simulink model "gyroYawLoop"  (R2015a)
settings: Solver=ode45  StartTime=0.0  StopTime=10  RelTol=1e-3
undefined symbols (not defined in the file or in its folder): dt, plantTorqueOffset, torqueOffset
libraries: simulink x1, vrlib x1
settings Model: Creator=johnz  LastModifiedBy=johnz

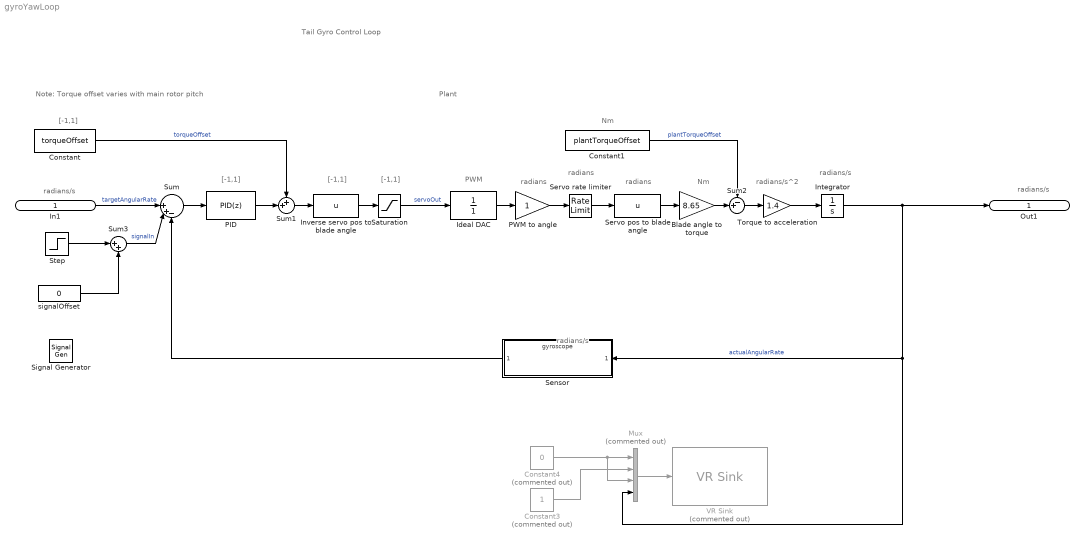
== system gyroYawLoop ==
  note: Tail Gyro Control Loop
  note: Note: Torque offset varies with main rotor pitch
  note: Plant
  note: [-1,1]
  note: radians/s
  note: radians
  note: radians/s^2
  note: radians/s
  note: [-1,1]
  note: [-1,1]
  note: [-1,1]
  note: Nm
  note: radians/s
  note: Nm
  note: radians
  note: radians
  note: radians/s
  note: PWM
  In1 : Inport  SampleTime=dt
  Blade angle to torque : Gain  Gain=8.65
  Constant : Constant  Value=torqueOffset  SampleTime=dt
  Constant1 : Constant  Value=plantTorqueOffset
  Constant3 : Constant  Commented=on
  Constant4 : Constant  Commented=on  Value=0
  Ideal DAC : TransferFcn  Denominator=[1]
  Integrator : Integrator
  "Inverse servo pos to blade angle " : Fcn  Expr=u
  Mux : Mux  Commented=on
  PID : simulink/Continuous/PID Controller  Controller=PID  TimeDomain=Discrete-time  SampleTime=dt  IntegratorMethod=Forward Euler  FilterMethod=Forward Euler  Form=Parallel  UseFilter=off  ControllerParametersSource=internal  P=1.08315527025018  I=2.38693404249782  D=.035  N=100  InitialConditionSource=internal  InitialConditionForIntegrator=0  InitialConditionForFilter=0  ExternalReset=none  ZeroCross=off  LimitOutput=on  UpperSaturationLimit=1 - torqueOffset  LowerSaturationLimit=-1 - torqueOffset  LinearizeAsGain=on  AntiWindupMode=clamping  Kb=0.5  TrackingMode=off  Kt=1  PParamMin=[]  PParamMax=[]  IParamMin=[]  IParamMax=[]  DParamMin=[]  DParamMax=[]  NParamMin=[]  NParamMax=[]  KbParamMin=[]  KbParamMax=[]  KtParamMin=[]  KtParamMax=[]  POutMin=[]  POutMax=[]  IOutMin=[]  IOutMax=[]  DOutMin=[]  DOutMax=[]  NOutMin=[]  NOutMax=[]  KbOutMin=[]  KbOutMax=[]  KtOutMin=[]  KtOutMax=[]  IntegratorOutMin=[]  IntegratorOutMax=[]  FilterOutMin=[]  FilterOutMax=[]  SumOutMin=[]  SumOutMax=[]  SumI1OutMin=[]  SumI1OutMax=[]  SumI2OutMin=[]  SumI2OutMax=[]  SumI3OutMin=[]  SumI3OutMax=[]  SumDOutMin=[]  SumDOutMax=[]  SaturationOutMin=[]  SaturationOutMax=[]  IntegratorContinuousStateAttributes=''  IntegratorStateMustResolveToSignalObject=off  IntegratorRTWStateStorageClass=Auto  FilterContinuousStateAttributes=''  FilterStateMustResolveToSignalObject=off  FilterRTWStateStorageClass=Auto  DifferentiatorICPrevScaledInput=0  DifferentiatorOutMin=[]  DifferentiatorOutMax=[]
  PWM to angle : Gain
  Saturation : Saturate  UpperLimit=1  LowerLimit=-1
  Sensor : ModelReference  ModelNameDialog=gyroscope.slx  ParameterArgumentNames=randomSeed  ParameterArgumentValues=1  SimulationMode=Normal  ModelReferenceVersion=1.23  CopyOfModelName=gyroscope.slx  DefaultDataLogging=on
  Servo pos to blade angle : Fcn  Expr=u
  Servo rate limiter : RateLimiter  RisingSlewLimit=15  FallingSlewLimit=-15  SampleTimeMode=inherited
  Signal Generator : SignalGenerator  WaveForm=square  Frequency=0.5  Units=rad/sec
  Step : Step  SampleTime=dt
  Sum : Sum  Inputs=||++-
  Sum1 : Sum  Inputs=++|
  Sum2 : Sum  Inputs=-+|
  Sum3 : Sum  Inputs=|++
  Torque to acceleration : Gain  Gain=1.4
  VR Sink : vrlib/VR Sink  Commented=on  InstantiateOnLoad=on  SampleTime=-1  ViewEnable=on  RemoteChange=off  RemoteView=off  FieldsWritten=Helicopter.rotation.4.1.1.double  WorldFileName=animation\animation_world.wrl  AutoView=off  VideoDimensions=[]  AllowVariableSize=off
  signalOffset : Constant  Value=0  SampleTime=dt
  Out1 : Outport
  wires:
  In1/1 -> Sum/1  "targetAngularRate"
  Servo rate limiter/1 -> Servo pos to blade angle/1
  Servo pos to blade angle/1 -> Blade angle to torque/1
  Constant/1 -> Sum1/1  "torqueOffset"
  Sum/1 -> PID/1
  Sum1/1 -> "Inverse servo pos to blade angle "/1
  "Inverse servo pos to blade angle "/1 -> Saturation/1
  Saturation/1 -> Ideal DAC/1  "servoOut"
  Torque to acceleration/1 -> Integrator/1
  Sum2/1 -> Torque to acceleration/1
  Blade angle to torque/1 -> Sum2/2
  Constant1/1 -> Sum2/1  "plantTorqueOffset"
  PWM to angle/1 -> Servo rate limiter/1
  signalOffset/1 -> Sum3/2
  Sum3/1 -> Sum/2  "signalIn"
  Integrator/1 -> Out1/1, Mux/4, Sensor/1  "actualAngularRate"
  Constant4/1 -> Mux/3, Mux/1
  Mux/1 -> VR Sink/1
  Constant3/1 -> Mux/2
  Ideal DAC/1 -> PWM to angle/1
  Step/1 -> Sum3/1
  PID/1 -> Sum1/2
  Sensor/1 -> Sum/3
